simulink model "Fly_By_Wire_Component_Architecture"  (R2025a)
settings: Solver=VariableStepAuto  StartTime=0.0  StopTime=10.0  RelTol=1e-3
settings Model: Creator=kmara  LastModifiedBy=annic

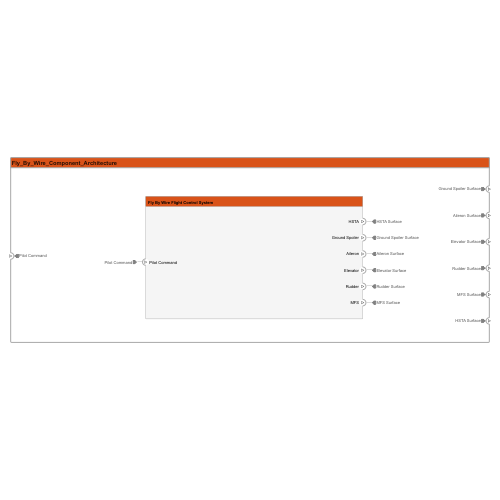
[thumbnail: Simulink's stored preview of the top-level diagram]
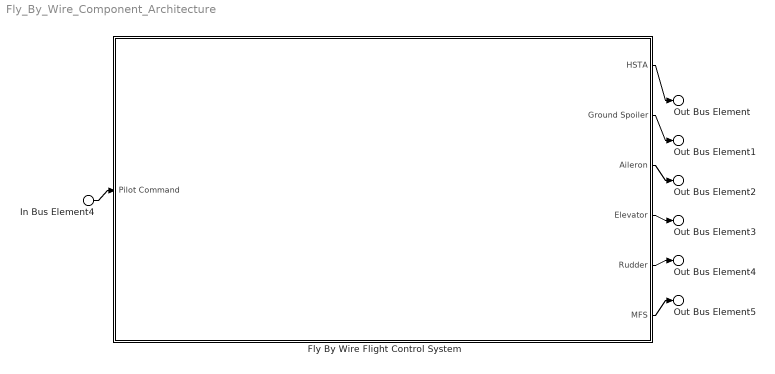
== system Fly_By_Wire_Component_Architecture ==
  In Bus Element4 : Inport  PortName=Pilot Command
  Fly By Wire Flight Control System : Subsystem
      settings: PortSchema="{\"entries\":[{\"content\":{\"headerSize\":26,\"margin\":15,\"minimumSpacing\":25,\"sides\":[{\"content\":{\"connectorIds\":[\"In1\"]},\"type\":\"ConnectorPlacement.EquallySpacedRectSide\",\"uuid\":\"7c02a101-dcdb-4ce7-aa42-618b1352dc14\"},{\"content\":{\"connectorIds\":[\"Out1\",\"Out2\",\"Out3\",\"Out4\",\"Out5\",\"Out6\"],\"side\":\"RIGHT\"},\"type\":\"ConnectorPlacement.EquallySpacedRectSide\",\"uuid\":\"7a5c8ca0-4377-40e0-b018-2d4752105c97\"},{\"content\":{\"side\":\"TOP\"},\"type\":\"ConnectorPlacement.EquallySpacedRectSide\",\"uuid\":\"1a585cfa-94cd-4fa4-8da7-05bff58353c8\"}]},\"type\":\"ConnectorPlacement.EquallySpacedConnector\",\"uuid\":\"b5a72803-1929-44a1-ac0b-19b19b30c1d3\"}],\"packageUris\":[\"http://schema.mathworks.com/mf0/Connector/R2020b\"],\"version\":\"1.0\"}"
  Out Bus Element1 : Outport  PortName=Ground Spoiler Surface
  Out Bus Element2 : Outport  Port=2  PortName=Aileron Surface
  Out Bus Element3 : Outport  Port=3  PortName=Elevator Surface
  Out Bus Element4 : Outport  Port=4  PortName=Rudder Surface
  Out Bus Element5 : Outport  Port=5  PortName=MFS Surface
  Out Bus Element : Outport  Port=6  PortName=HSTA Surface
  wires:
  Fly By Wire Flight Control System/1(HSTA) -> Out Bus Element/1
  Fly By Wire Flight Control System/2(Ground Spoiler) -> Out Bus Element1/1
  Fly By Wire Flight Control System/3(Aileron) -> Out Bus Element2/1
  Fly By Wire Flight Control System/4(Elevator) -> Out Bus Element3/1
  Fly By Wire Flight Control System/5(Rudder) -> Out Bus Element4/1
  Fly By Wire Flight Control System/6(MFS) -> Out Bus Element5/1
  In Bus Element4/1 -> Fly By Wire Flight Control System/1(Pilot Command)

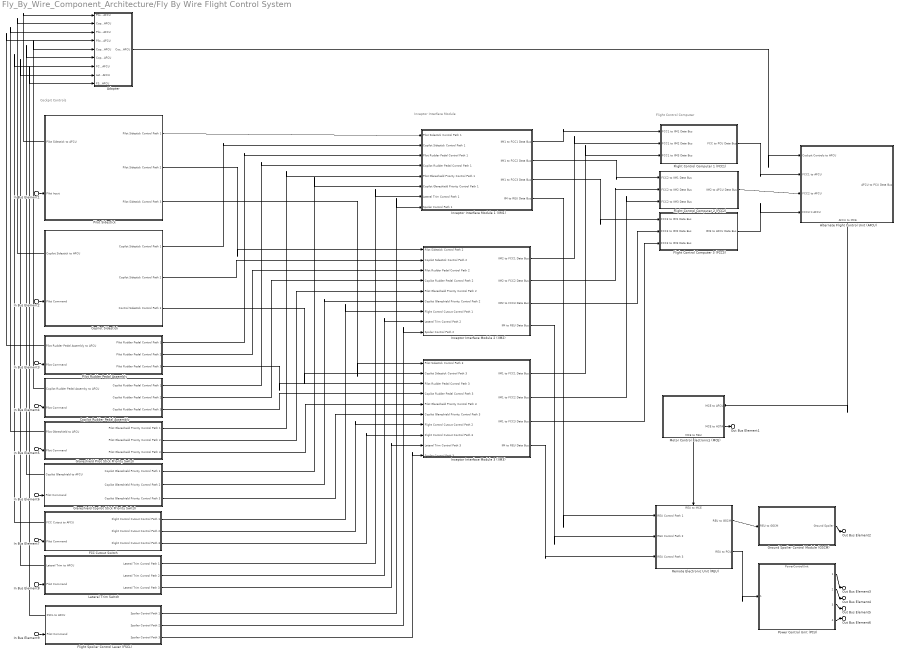
== system Fly_By_Wire_Component_Architecture/Fly By Wire Flight Control System ==
  note: Inceptor Interface Module
  note: Flight Control Computer
  note: Cockpit Controls
  In Bus Element{1..9} (9 alike) : Inport  PortName=Pilot Command
  Adapter : Subsystem
      settings: PortSchema="{\"entries\":[{\"content\":{\"margin\":10,\"minimumSpacing\":15,\"sides\":[{\"content\":{\"connectorIds\":[\"In9\",\"In2\",\"In1\",\"In3\",\"In4\",\"In5\",\"In6\",\"In7\",\"In8\"]},\"type\":\"ConnectorPlacement.EquallySpacedRectSide\",\"uuid\":\"7c02a101-dcdb-4ce7-aa42-618b1352dc14\"},{\"content\":{\"connectorIds\":[\"Out1\"],\"side\":\"RIGHT\"},\"type\":\"ConnectorPlacement.EquallySpacedRectSide\",\"uuid\":\"7a5c8ca0-4377-40e0-b018-2d4752105c97\"},{\"content\":{\"side\":\"TOP\"},\"type\":\"ConnectorPlacement.EquallySpacedRectSide\",\"uuid\":\"1a585cfa-94cd-4fa4-8da7-05bff58353c8\"},{\"content\":{\"side\":\"BOTTOM\"},\"type\":\"ConnectorPlacement.EquallySpacedRectSide\",\"uuid\":\"bc495dab-060b-4ff9-9574-e388694fe188\"}]},\"type\":\"ConnectorPlacement.EquallySpacedConnector\",\"uuid\":\"b5a72803-1929-44a1-ac0b-19b19b30c1d3\"}],\"packageUris\":[\"http://schema.mathworks.com/mf0/Connector/R2020b\"],\"version\":\"1.0\"}"
  Alternate Flight Control Unit (AFCU) : Subsystem
      settings: PortSchema="{\"entries\":[{\"content\":{\"headerSize\":26,\"margin\":15,\"minimumSpacing\":25,\"sides\":[{\"content\":{\"connectorIds\":[\"In1\",\"In2\",\"In3\",\"In4\"]},\"type\":\"ConnectorPlacement.EquallySpacedRectSide\",\"uuid\":\"76a6f17d-cf4a-44f4-8892-601f52e19bd9\"},{\"content\":{\"connectorIds\":[\"Out2\"],\"side\":\"RIGHT\"},\"type\":\"ConnectorPlacement.EquallySpacedRectSide\",\"uuid\":\"5dcbb71c-e863-4861-a43d-ad9fb4188728\"},{\"content\":{\"side\":\"TOP\"},\"type\":\"ConnectorPlacement.EquallySpacedRectSide\",\"uuid\":\"68738236-1483-402e-9d85-5d65cc06fd90\"},{\"content\":{\"connectorIds\":[\"Out1\"],\"side\":\"BOTTOM\"},\"type\":\"ConnectorPlacement.EquallySpacedRectSide\",\"uuid\":\"9a083ef4-6723-4d8e-ad60-e307f1dd41e6\"}]},\"type\":\"ConnectorPlacement.EquallySpacedConnector\",\"uuid\":\"56deb81c-b974-4059-9f73-f14d44365067\"}],\"packageUris\":[\"http://schema.mathworks.com/mf0/Connector/R2020b\"],\"version\":\"1.0\"}"
  Copilot Rudder Pedal Assembly : Subsystem
      settings: PortSchema="{\"entries\":[{\"content\":{\"headerSize\":26,\"margin\":15,\"minimumSpacing\":25,\"sides\":[{\"content\":{\"connectorIds\":[\"Out1\",\"In1\"]},\"type\":\"ConnectorPlacement.EquallySpacedRectSide\",\"uuid\":\"76a6f17d-cf4a-44f4-8892-601f52e19bd9\"},{\"content\":{\"connectorIds\":[\"Out2\",\"Out3\",\"Out4\"],\"side\":\"RIGHT\"},\"type\":\"ConnectorPlacement.EquallySpacedRectSide\",\"uuid\":\"5dcbb71c-e863-4861-a43d-ad9fb4188728\"},{\"content\":{\"side\":\"TOP\"},\"type\":\"ConnectorPlacement.EquallySpacedRectSide\",\"uuid\":\"68738236-1483-402e-9d85-5d65cc06fd90\"}]},\"type\":\"ConnectorPlacement.EquallySpacedConnector\",\"uuid\":\"56deb81c-b974-4059-9f73-f14d44365067\"}],\"packageUris\":[\"http://schema.mathworks.com/mf0/Connector/R2020b\"],\"version\":\"1.0\"}"
  Copilot Sidestick : Subsystem
      settings: PortSchema="{\"entries\":[{\"content\":{\"headerSize\":26,\"margin\":15,\"minimumSpacing\":25,\"sides\":[{\"content\":{\"connectorIds\":[\"Out1\",\"In1\"]},\"type\":\"ConnectorPlacement.EquallySpacedRectSide\",\"uuid\":\"76a6f17d-cf4a-44f4-8892-601f52e19bd9\"},{\"content\":{\"connectorIds\":[\"Out2\",\"Out3\",\"Out4\"],\"side\":\"RIGHT\"},\"type\":\"ConnectorPlacement.EquallySpacedRectSide\",\"uuid\":\"5dcbb71c-e863-4861-a43d-ad9fb4188728\"},{\"content\":{\"side\":\"TOP\"},\"type\":\"ConnectorPlacement.EquallySpacedRectSide\",\"uuid\":\"68738236-1483-402e-9d85-5d65cc06fd90\"}]},\"type\":\"ConnectorPlacement.EquallySpacedConnector\",\"uuid\":\"56deb81c-b974-4059-9f73-f14d44365067\"}],\"packageUris\":[\"http://schema.mathworks.com/mf0/Connector/R2020b\"],\"version\":\"1.0\"}"
  FCC Cutout Switch : Subsystem
      settings: PortSchema="{\"entries\":[{\"content\":{\"headerSize\":26,\"margin\":15,\"minimumSpacing\":25,\"sides\":[{\"content\":{\"connectorIds\":[\"Out1\",\"In1\"]},\"type\":\"ConnectorPlacement.EquallySpacedRectSide\",\"uuid\":\"76a6f17d-cf4a-44f4-8892-601f52e19bd9\"},{\"content\":{\"connectorIds\":[\"Out2\",\"Out3\",\"Out4\"],\"side\":\"RIGHT\"},\"type\":\"ConnectorPlacement.EquallySpacedRectSide\",\"uuid\":\"5dcbb71c-e863-4861-a43d-ad9fb4188728\"},{\"content\":{\"side\":\"TOP\"},\"type\":\"ConnectorPlacement.EquallySpacedRectSide\",\"uuid\":\"68738236-1483-402e-9d85-5d65cc06fd90\"}]},\"type\":\"ConnectorPlacement.EquallySpacedConnector\",\"uuid\":\"56deb81c-b974-4059-9f73-f14d44365067\"}],\"packageUris\":[\"http://schema.mathworks.com/mf0/Connector/R2020b\"],\"version\":\"1.0\"}"
  Flight Control Computer 1 (FCC1) : Subsystem
      settings: PortSchema="{\"entries\":[{\"content\":{\"headerSize\":26,\"margin\":15,\"minimumSpacing\":25,\"sides\":[{\"content\":{\"connectorIds\":[\"In1\",\"In2\",\"In3\"]},\"type\":\"ConnectorPlacement.EquallySpacedRectSide\",\"uuid\":\"76a6f17d-cf4a-44f4-8892-601f52e19bd9\"},{\"content\":{\"connectorIds\":[\"Out1\"],\"side\":\"RIGHT\"},\"type\":\"ConnectorPlacement.EquallySpacedRectSide\",\"uuid\":\"5dcbb71c-e863-4861-a43d-ad9fb4188728\"},{\"content\":{\"side\":\"TOP\"},\"type\":\"ConnectorPlacement.EquallySpacedRectSide\",\"uuid\":\"68738236-1483-402e-9d85-5d65cc06fd90\"}]},\"type\":\"ConnectorPlacement.EquallySpacedConnector\",\"uuid\":\"56deb81c-b974-4059-9f73-f14d44365067\"}],\"packageUris\":[\"http://schema.mathworks.com/mf0/Connector/R2020b\"],\"version\":\"1.0\"}"
  Flight Control Computer 2 (FCC2) : Subsystem
      settings: PortSchema="{\"entries\":[{\"content\":{\"headerSize\":26,\"margin\":15,\"minimumSpacing\":25,\"sides\":[{\"content\":{\"connectorIds\":[\"In1\",\"In2\",\"In3\"]},\"type\":\"ConnectorPlacement.EquallySpacedRectSide\",\"uuid\":\"3265125f-5582-4687-bb7d-dadd2bb28ee5\"},{\"content\":{\"connectorIds\":[\"Out1\"],\"side\":\"RIGHT\"},\"type\":\"ConnectorPlacement.EquallySpacedRectSide\",\"uuid\":\"e765b43a-7d93-4967-9a71-e180bcccebcf\"},{\"content\":{\"side\":\"TOP\"},\"type\":\"ConnectorPlacement.EquallySpacedRectSide\",\"uuid\":\"6eb4b4e6-82d4-477f-9521-c512acf3f79c\"}]},\"type\":\"ConnectorPlacement.EquallySpacedConnector\",\"uuid\":\"cacda304-df90-44d5-b969-56e5837c68bb\"}],\"packageUris\":[\"http://schema.mathworks.com/mf0/Connector/R2020b\"],\"version\":\"1.0\"}"
  Flight Control Computer 3 (FCC3) : Subsystem
      settings: PortSchema="{\"entries\":[{\"content\":{\"headerSize\":26,\"margin\":15,\"minimumSpacing\":25,\"sides\":[{\"content\":{\"connectorIds\":[\"In1\",\"In2\",\"In3\"]},\"type\":\"ConnectorPlacement.EquallySpacedRectSide\",\"uuid\":\"3265125f-5582-4687-bb7d-dadd2bb28ee5\"},{\"content\":{\"connectorIds\":[\"Out1\"],\"side\":\"RIGHT\"},\"type\":\"ConnectorPlacement.EquallySpacedRectSide\",\"uuid\":\"e765b43a-7d93-4967-9a71-e180bcccebcf\"},{\"content\":{\"side\":\"TOP\"},\"type\":\"ConnectorPlacement.EquallySpacedRectSide\",\"uuid\":\"6eb4b4e6-82d4-477f-9521-c512acf3f79c\"}]},\"type\":\"ConnectorPlacement.EquallySpacedConnector\",\"uuid\":\"cacda304-df90-44d5-b969-56e5837c68bb\"}],\"packageUris\":[\"http://schema.mathworks.com/mf0/Connector/R2020b\"],\"version\":\"1.0\"}"
  Flight Spoiler Control Lever (FSCL) : Subsystem
      settings: PortSchema="{\"entries\":[{\"content\":{\"headerSize\":26,\"margin\":15,\"minimumSpacing\":25,\"sides\":[{\"content\":{\"connectorIds\":[\"Out1\",\"In1\"]},\"type\":\"ConnectorPlacement.EquallySpacedRectSide\",\"uuid\":\"76a6f17d-cf4a-44f4-8892-601f52e19bd9\"},{\"content\":{\"connectorIds\":[\"Out2\",\"Out3\",\"Out4\"],\"side\":\"RIGHT\"},\"type\":\"ConnectorPlacement.EquallySpacedRectSide\",\"uuid\":\"5dcbb71c-e863-4861-a43d-ad9fb4188728\"},{\"content\":{\"side\":\"TOP\"},\"type\":\"ConnectorPlacement.EquallySpacedRectSide\",\"uuid\":\"68738236-1483-402e-9d85-5d65cc06fd90\"}]},\"type\":\"ConnectorPlacement.EquallySpacedConnector\",\"uuid\":\"56deb81c-b974-4059-9f73-f14d44365067\"}],\"packageUris\":[\"http://schema.mathworks.com/mf0/Connector/R2020b\"],\"version\":\"1.0\"}"
  Glareshield Copilot Stick Priority Switch : Subsystem
      settings: PortSchema="{\"entries\":[{\"content\":{\"headerSize\":26,\"margin\":15,\"minimumSpacing\":25,\"sides\":[{\"content\":{\"connectorIds\":[\"Out1\",\"In1\"]},\"type\":\"ConnectorPlacement.EquallySpacedRectSide\",\"uuid\":\"76a6f17d-cf4a-44f4-8892-601f52e19bd9\"},{\"content\":{\"connectorIds\":[\"Out2\",\"Out3\",\"Out4\"],\"side\":\"RIGHT\"},\"type\":\"ConnectorPlacement.EquallySpacedRectSide\",\"uuid\":\"5dcbb71c-e863-4861-a43d-ad9fb4188728\"},{\"content\":{\"side\":\"TOP\"},\"type\":\"ConnectorPlacement.EquallySpacedRectSide\",\"uuid\":\"68738236-1483-402e-9d85-5d65cc06fd90\"}]},\"type\":\"ConnectorPlacement.EquallySpacedConnector\",\"uuid\":\"56deb81c-b974-4059-9f73-f14d44365067\"}],\"packageUris\":[\"http://schema.mathworks.com/mf0/Connector/R2020b\"],\"version\":\"1.0\"}"
  Glareshield Pilot Stick Priority Switch : Subsystem
      settings: PortSchema="{\"entries\":[{\"content\":{\"headerSize\":26,\"margin\":15,\"minimumSpacing\":25,\"sides\":[{\"content\":{\"connectorIds\":[\"Out1\",\"In1\"]},\"type\":\"ConnectorPlacement.EquallySpacedRectSide\",\"uuid\":\"76a6f17d-cf4a-44f4-8892-601f52e19bd9\"},{\"content\":{\"connectorIds\":[\"Out2\",\"Out3\",\"Out4\"],\"side\":\"RIGHT\"},\"type\":\"ConnectorPlacement.EquallySpacedRectSide\",\"uuid\":\"5dcbb71c-e863-4861-a43d-ad9fb4188728\"},{\"content\":{\"side\":\"TOP\"},\"type\":\"ConnectorPlacement.EquallySpacedRectSide\",\"uuid\":\"68738236-1483-402e-9d85-5d65cc06fd90\"}]},\"type\":\"ConnectorPlacement.EquallySpacedConnector\",\"uuid\":\"56deb81c-b974-4059-9f73-f14d44365067\"}],\"packageUris\":[\"http://schema.mathworks.com/mf0/Connector/R2020b\"],\"version\":\"1.0\"}"
  Ground Spoiler Control Module (GSCM) : Subsystem
      settings: PortSchema="{\"entries\":[{\"content\":{\"headerSize\":26,\"margin\":15,\"minimumSpacing\":25,\"sides\":[{\"content\":{\"connectorIds\":[\"In1\"]},\"type\":\"ConnectorPlacement.EquallySpacedRectSide\",\"uuid\":\"76a6f17d-cf4a-44f4-8892-601f52e19bd9\"},{\"content\":{\"connectorIds\":[\"Out1\"],\"side\":\"RIGHT\"},\"type\":\"ConnectorPlacement.EquallySpacedRectSide\",\"uuid\":\"5dcbb71c-e863-4861-a43d-ad9fb4188728\"},{\"content\":{\"side\":\"TOP\"},\"type\":\"ConnectorPlacement.EquallySpacedRectSide\",\"uuid\":\"68738236-1483-402e-9d85-5d65cc06fd90\"}]},\"type\":\"ConnectorPlacement.EquallySpacedConnector\",\"uuid\":\"56deb81c-b974-4059-9f73-f14d44365067\"}],\"packageUris\":[\"http://schema.mathworks.com/mf0/Connector/R2020b\"],\"version\":\"1.0\"}"
  Inceptor Interface Module 1 (IIM1) : Subsystem
      settings: PortSchema="{\"entries\":[{\"content\":{\"headerSize\":26,\"margin\":15,\"minimumSpacing\":25,\"sides\":[{\"content\":{\"connectorIds\":[\"In1\",\"In2\",\"In3\",\"In4\",\"In5\",\"In6\",\"In7\",\"In8\"]},\"type\":\"ConnectorPlacement.EquallySpacedRectSide\",\"uuid\":\"76a6f17d-cf4a-44f4-8892-601f52e19bd9\"},{\"content\":{\"connectorIds\":[\"Out1\",\"Out2\",\"Out3\",\"Out4\"],\"side\":\"RIGHT\"},\"type\":\"ConnectorPlacement.EquallySpacedRectSide\",\"uuid\":\"5dcbb71c-e863-4861-a43d-ad9fb4188728\"},{\"content\":{\"side\":\"TOP\"},\"type\":\"ConnectorPlacement.EquallySpacedRectSide\",\"uuid\":\"68738236-1483-402e-9d85-5d65cc06fd90\"},{\"content\":{\"side\":\"BOTTOM\"},\"type\":\"ConnectorPlacement.EquallySpacedRectSide\",\"uuid\":\"f9a83800-3852-40cb-9c1f-6e0812a46961\"}]},\"type\":\"ConnectorPlacement.EquallySpacedConnector\",\"uuid\":\"56deb81c-b974-4059-9f73-f14d44365067\"}],\"packageUris\":[\"http://schema.mathworks.com/mf0/Connector/R2020b\"],\"version\":\"1.0\"}"
  Inceptor Interface Module 2 (IIM2) : Subsystem
      settings: PortSchema="{\"entries\":[{\"content\":{\"headerSize\":26,\"margin\":15,\"minimumSpacing\":25,\"sides\":[{\"content\":{\"connectorIds\":[\"In1\",\"In3\",\"In2\",\"In4\",\"In5\",\"In6\",\"In7\",\"In8\",\"In9\"]},\"type\":\"ConnectorPlacement.EquallySpacedRectSide\",\"uuid\":\"76a6f17d-cf4a-44f4-8892-601f52e19bd9\"},{\"content\":{\"connectorIds\":[\"Out1\",\"Out2\",\"Out3\",\"Out4\"],\"side\":\"RIGHT\"},\"type\":\"ConnectorPlacement.EquallySpacedRectSide\",\"uuid\":\"5dcbb71c-e863-4861-a43d-ad9fb4188728\"},{\"content\":{\"side\":\"TOP\"},\"type\":\"ConnectorPlacement.EquallySpacedRectSide\",\"uuid\":\"68738236-1483-402e-9d85-5d65cc06fd90\"},{\"content\":{\"side\":\"BOTTOM\"},\"type\":\"ConnectorPlacement.EquallySpacedRectSide\",\"uuid\":\"f9a83800-3852-40cb-9c1f-6e0812a46961\"}]},\"type\":\"ConnectorPlacement.EquallySpacedConnector\",\"uuid\":\"56deb81c-b974-4059-9f73-f14d44365067\"}],\"packageUris\":[\"http://schema.mathworks.com/mf0/Connector/R2020b\"],\"version\":\"1.0\"}"
  Inceptor Interface Module 3 (IIM3) : Subsystem
      settings: PortSchema="{\"entries\":[{\"content\":{\"headerSize\":26,\"margin\":15,\"minimumSpacing\":25,\"sides\":[{\"content\":{\"connectorIds\":[\"In1\",\"In2\",\"In3\",\"In4\",\"In5\",\"In6\",\"In7\",\"In8\",\"In9\",\"In10\"]},\"type\":\"ConnectorPlacement.EquallySpacedRectSide\",\"uuid\":\"76a6f17d-cf4a-44f4-8892-601f52e19bd9\"},{\"content\":{\"connectorIds\":[\"Out1\",\"Out2\",\"Out3\",\"Out4\"],\"side\":\"RIGHT\"},\"type\":\"ConnectorPlacement.EquallySpacedRectSide\",\"uuid\":\"5dcbb71c-e863-4861-a43d-ad9fb4188728\"},{\"content\":{\"side\":\"TOP\"},\"type\":\"ConnectorPlacement.EquallySpacedRectSide\",\"uuid\":\"68738236-1483-402e-9d85-5d65cc06fd90\"},{\"content\":{\"side\":\"BOTTOM\"},\"type\":\"ConnectorPlacement.EquallySpacedRectSide\",\"uuid\":\"f9a83800-3852-40cb-9c1f-6e0812a46961\"}]},\"type\":\"ConnectorPlacement.EquallySpacedConnector\",\"uuid\":\"56deb81c-b974-4059-9f73-f14d44365067\"}],\"packageUris\":[\"http://schema.mathworks.com/mf0/Connector/R2020b\"],\"version\":\"1.0\"}"
  Lateral Trim Switch : Subsystem
      settings: PortSchema="{\"entries\":[{\"content\":{\"headerSize\":26,\"margin\":15,\"minimumSpacing\":25,\"sides\":[{\"content\":{\"connectorIds\":[\"Out1\",\"In1\"]},\"type\":\"ConnectorPlacement.EquallySpacedRectSide\",\"uuid\":\"76a6f17d-cf4a-44f4-8892-601f52e19bd9\"},{\"content\":{\"connectorIds\":[\"Out2\",\"Out3\",\"Out4\"],\"side\":\"RIGHT\"},\"type\":\"ConnectorPlacement.EquallySpacedRectSide\",\"uuid\":\"5dcbb71c-e863-4861-a43d-ad9fb4188728\"},{\"content\":{\"side\":\"TOP\"},\"type\":\"ConnectorPlacement.EquallySpacedRectSide\",\"uuid\":\"68738236-1483-402e-9d85-5d65cc06fd90\"}]},\"type\":\"ConnectorPlacement.EquallySpacedConnector\",\"uuid\":\"56deb81c-b974-4059-9f73-f14d44365067\"}],\"packageUris\":[\"http://schema.mathworks.com/mf0/Connector/R2020b\"],\"version\":\"1.0\"}"
  Motor Control Electronics (MCE) : Subsystem
      settings: PortSchema="{\"entries\":[{\"content\":{\"headerSize\":26,\"margin\":15,\"minimumSpacing\":25,\"sides\":[{\"content\":{},\"type\":\"ConnectorPlacement.EquallySpacedRectSide\",\"uuid\":\"7c02a101-dcdb-4ce7-aa42-618b1352dc14\"},{\"content\":{\"connectorIds\":[\"In1\",\"Out1\"],\"side\":\"RIGHT\"},\"type\":\"ConnectorPlacement.EquallySpacedRectSide\",\"uuid\":\"7a5c8ca0-4377-40e0-b018-2d4752105c97\"},{\"content\":{\"side\":\"TOP\"},\"type\":\"ConnectorPlacement.EquallySpacedRectSide\",\"uuid\":\"1a585cfa-94cd-4fa4-8da7-05bff58353c8\"},{\"content\":{\"connectorIds\":[\"Out2\"],\"side\":\"BOTTOM\"},\"type\":\"ConnectorPlacement.EquallySpacedRectSide\",\"uuid\":\"a4e30391-3178-49c1-81f8-9566370a7e69\"}]},\"type\":\"ConnectorPlacement.EquallySpacedConnector\",\"uuid\":\"b5a72803-1929-44a1-ac0b-19b19b30c1d3\"}],\"packageUris\":[\"http://schema.mathworks.com/mf0/Connector/R2020b\"],\"version\":\"1.0\"}"
  Pilot Rudder Pedal Assembly : Subsystem
      settings: PortSchema="{\"entries\":[{\"content\":{\"headerSize\":26,\"margin\":15,\"minimumSpacing\":25,\"sides\":[{\"content\":{\"connectorIds\":[\"Out1\",\"In1\"]},\"type\":\"ConnectorPlacement.EquallySpacedRectSide\",\"uuid\":\"76a6f17d-cf4a-44f4-8892-601f52e19bd9\"},{\"content\":{\"connectorIds\":[\"Out2\",\"Out4\",\"Out3\"],\"side\":\"RIGHT\"},\"type\":\"ConnectorPlacement.EquallySpacedRectSide\",\"uuid\":\"5dcbb71c-e863-4861-a43d-ad9fb4188728\"},{\"content\":{\"side\":\"TOP\"},\"type\":\"ConnectorPlacement.EquallySpacedRectSide\",\"uuid\":\"68738236-1483-402e-9d85-5d65cc06fd90\"}]},\"type\":\"ConnectorPlacement.EquallySpacedConnector\",\"uuid\":\"56deb81c-b974-4059-9f73-f14d44365067\"}],\"packageUris\":[\"http://schema.mathworks.com/mf0/Connector/R2020b\"],\"version\":\"1.0\"}"
  Pilot Sidestick : Subsystem
      settings: PortSchema="{\"entries\":[{\"content\":{\"headerSize\":26,\"margin\":15,\"minimumSpacing\":25,\"sides\":[{\"content\":{\"connectorIds\":[\"Out4\",\"In1\"]},\"type\":\"ConnectorPlacement.EquallySpacedRectSide\",\"uuid\":\"76a6f17d-cf4a-44f4-8892-601f52e19bd9\"},{\"content\":{\"connectorIds\":[\"Out1\",\"Out2\",\"Out3\"],\"side\":\"RIGHT\"},\"type\":\"ConnectorPlacement.EquallySpacedRectSide\",\"uuid\":\"5dcbb71c-e863-4861-a43d-ad9fb4188728\"},{\"content\":{\"side\":\"TOP\"},\"type\":\"ConnectorPlacement.EquallySpacedRectSide\",\"uuid\":\"68738236-1483-402e-9d85-5d65cc06fd90\"}]},\"type\":\"ConnectorPlacement.EquallySpacedConnector\",\"uuid\":\"56deb81c-b974-4059-9f73-f14d44365067\"}],\"packageUris\":[\"http://schema.mathworks.com/mf0/Connector/R2020b\"],\"version\":\"1.0\"}"
  Power Control Unit (PCU) : ModelReference  ModelNameDialog=PowerControlUnit  SimulationMode=Normal  ModelReferenceVersion=3.0
      settings: PortSchema="{\"entries\":[{\"content\":{\"headerSize\":38,\"margin\":15,\"minimumSpacing\":25,\"sides\":[{\"content\":{\"connectorIds\":[\"In1\"]},\"type\":\"ConnectorPlacement.EquallySpacedRectSide\",\"uuid\":\"b5cc4046-2a7b-4e82-a24e-8f0b5fbe8f3b\"},{\"content\":{\"connectorIds\":[\"Out1\",\"Out2\",\"Out3\",\"Out4\"],\"side\":\"RIGHT\"},\"type\":\"ConnectorPlacement.EquallySpacedRectSide\",\"uuid\":\"a37fb25c-992f-4dee-9f4d-cb05ec6d06aa\"},{\"content\":{\"side\":\"TOP\"},\"type\":\"ConnectorPlacement.EquallySpacedRectSide\",\"uuid\":\"6865807b-cb28-45bc-8645-e4c4882f3eb7\"}]},\"type\":\"ConnectorPlacement.EquallySpacedConnector\",\"uuid\":\"a108b503-ea1d-46cf-b1fa-be423a2d8416\"}],\"packageUris\":[\"http://schema.mathworks.com/mf0/Connector/R2020b\"],\"version\":\"1.0\"}"
  Remote Electronic Unit (REU) : Subsystem
      settings: PortSchema="{\"entries\":[{\"content\":{\"headerSize\":26,\"margin\":15,\"minimumSpacing\":25,\"sides\":[{\"content\":{\"connectorIds\":[\"In2\",\"In3\",\"In4\"]},\"type\":\"ConnectorPlacement.EquallySpacedRectSide\",\"uuid\":\"76a6f17d-cf4a-44f4-8892-601f52e19bd9\"},{\"content\":{\"connectorIds\":[\"Out1\",\"Out2\"],\"side\":\"RIGHT\"},\"type\":\"ConnectorPlacement.EquallySpacedRectSide\",\"uuid\":\"5dcbb71c-e863-4861-a43d-ad9fb4188728\"},{\"content\":{\"connectorIds\":[\"In1\"],\"side\":\"TOP\"},\"type\":\"ConnectorPlacement.EquallySpacedRectSide\",\"uuid\":\"68738236-1483-402e-9d85-5d65cc06fd90\"},{\"content\":{\"side\":\"BOTTOM\"},\"type\":\"ConnectorPlacement.EquallySpacedRectSide\",\"uuid\":\"ca264cd1-95f3-4bee-bece-6d79b6f7bd38\"}]},\"type\":\"ConnectorPlacement.EquallySpacedConnector\",\"uuid\":\"56deb81c-b974-4059-9f73-f14d44365067\"}],\"packageUris\":[\"http://schema.mathworks.com/mf0/Connector/R2020b\"],\"version\":\"1.0\"}"
  Out Bus Element1 : Outport  PortName=HSTA
  Out Bus Element2 : Outport  Port=2  PortName=Ground Spoiler
  Out Bus Element3 : Outport  Port=3  PortName=Aileron
  Out Bus Element4 : Outport  Port=4  PortName=Elevator
  Out Bus Element5 : Outport  Port=5  PortName=Rudder
  Out Bus Element6 : Outport  Port=6  PortName=MFS
  wires:
  In Bus Element7/1 -> FCC Cutout Switch/1(Pilot Command)
  In Bus Element2/1 -> Copilot Sidestick/1(Pilot Command)
  Motor Control Electronics (MCE)/1(MCE to HSTA) -> Out Bus Element1/1
  Alternate Flight Control Unit (AFCU)/1(AFCU to MCE) -> Motor Control Electronics (MCE)/1(MCE to AFCU)
  Motor Control Electronics (MCE)/2(MCE to REU) -> Remote Electronic Unit (REU)/1(REU to MCE)
  FCC Cutout Switch/1(FCC Cutout to AFCU) -> Adapter/6(FCC Cutout to AFCU)
  Flight Spoiler Control Lever (FSCL)/1(FSCL to AFCU) -> Adapter/8(FSCL to AFCU)
  Remote Electronic Unit (REU)/1(REU to GSCM) -> Ground Spoiler Control Module (GSCM)/1(REU to GSCM)
  Pilot Sidestick/1(Pilot Sidestick Control Path 1) -> Inceptor Interface Module 1 (IIM1)/1(Pilot Sidestick Control Path 1)
  Ground Spoiler Control Module (GSCM)/1(Ground Spoiler) -> Out Bus Element2/1
  Copilot Rudder Pedal Assembly/3(Copilot Rudder Pedal Control Path 2) -> Inceptor Interface Module 2 (IIM2)/4(Copilot Rudder Pedal Control Path 2)
  Lateral Trim Switch/1(Lateral Trim to AFCU) -> Adapter/7(Lateral Trim to AFCU)
  Flight Control Computer 1 (FCC1)/1(FCC to PCU Data Bus) -> Alternate Flight Control Unit (AFCU)/2(FCC1 to AFCU)
  In Bus Element9/1 -> Flight Spoiler Control Lever (FSCL)/1(Pilot Command)
  FCC Cutout Switch/2(Flight Control Cutout Control Path 1) -> Inceptor Interface Module 2 (IIM2)/7(Flight Control Cutout Control Path 1)
  Lateral Trim Switch/3(Lateral Trim Control Path 2) -> Inceptor Interface Module 2 (IIM2)/8(Lateral Trim Control Path 2)
  Inceptor Interface Module 3 (IIM3)/2(IIM1 to FCC2 Data Bus) -> Flight Control Computer 2 (FCC2)/3(FCC2 to IIM3 Data Bus)
  Pilot Sidestick/2("Pilot Sidestick Control Path 2 ") -> Inceptor Interface Module 2 (IIM2)/1("Pilot Sidestick Control Path 2 ")
  Glareshield Copilot Stick Priority Switch/2(Copilot Glareshield Priority Control Path 1) -> Inceptor Interface Module 1 (IIM1)/6(Copilot Glareshield Priority Control Path 1)
  Flight Spoiler Control Lever (FSCL)/2(Spoiler Control Path 1) -> Inceptor Interface Module 1 (IIM1)/8(Spoiler Control Path 1)
  Pilot Sidestick/3(Pilot Sidestick Control Path 3) -> Inceptor Interface Module 3 (IIM3)/1("Pilot Sidestick Control Path 3 ")
  Flight Control Computer 2 (FCC2)/1(IIM2 to AFCU Data Bus) -> Alternate Flight Control Unit (AFCU)/3(FCC2 to AFCU)
  Lateral Trim Switch/4(Lateral Trim Control Path 3) -> Inceptor Interface Module 3 (IIM3)/9(Lateral Trim Control Path 3)
  Pilot Rudder Pedal Assembly/4(Pilot Rudder Pedal Control Path 2) -> Inceptor Interface Module 2 (IIM2)/2(Pilot Rudder Pedal Control Path 2)
  Copilot Sidestick/2(Copilot Sidestick Control Path 1) -> Inceptor Interface Module 1 (IIM1)/2(Copilot Sidestick Control Path 1)
  Glareshield Copilot Stick Priority Switch/4(Copilot Glareshield Priority Control Path 3) -> Inceptor Interface Module 3 (IIM3)/6(Copilot Glareshield Priority Control Path 3)
  Glareshield Copilot Stick Priority Switch/3(Copilot Glareshield Priority Control Path 2) -> Inceptor Interface Module 2 (IIM2)/6(Copilot Glareshield Priority Control Path 2)
  Glareshield Pilot Stick Priority Switch/3(Pilot Glareshield Priority Control Path 2) -> Inceptor Interface Module 2 (IIM2)/5(Pilot Glareshield Priority Control Path 2)
  Flight Spoiler Control Lever (FSCL)/4(Spoiler Control Path 3) -> Inceptor Interface Module 3 (IIM3)/10(Spoiler Control Path 3)
  Inceptor Interface Module 1 (IIM1)/2(IIM1 to FCC2 Data Bus) -> Flight Control Computer 2 (FCC2)/1(FCC2 to IIM1 Data Bus)
  Inceptor Interface Module 2 (IIM2)/1(IIM2 to FCC1 Data Bus) -> Flight Control Computer 1 (FCC1)/2(FCC1 to IIM2 Data Bus)
  Inceptor Interface Module 1 (IIM1)/3(IIM1 to FCC3 Data Bus) -> Flight Control Computer 3 (FCC3)/1(FCC3 to IIM1 Data Bus)
  Pilot Rudder Pedal Assembly/2(Pilot Rudder Pedal Control Path 1) -> Inceptor Interface Module 1 (IIM1)/3(Pilot Rudder Pedal Control Path 1)
  Copilot Sidestick/4(Control Sidestick Control Path 3) -> Inceptor Interface Module 3 (IIM3)/2(Copilot Sidestick Control Path 3)
  Inceptor Interface Module 1 (IIM1)/1(IIM1 to FCC1 Data Bus) -> Flight Control Computer 1 (FCC1)/1(FCC1 to IIM1 Data Bus)
  Copilot Sidestick/1(Copilot Sidestick to AFCU) -> Adapter/2(Copilot Sidestick to AFCU)
  FCC Cutout Switch/3(Flight Control Cutout Control Path 2) -> Inceptor Interface Module 3 (IIM3)/7(Flight Control Cutout Control Path 2)
  Inceptor Interface Module 2 (IIM2)/4(IIM to REU Data Bus) -> Remote Electronic Unit (REU)/3(REU Control Path 2)
  Flight Spoiler Control Lever (FSCL)/3(Spoiler Control Path 2) -> Inceptor Interface Module 2 (IIM2)/9(Spoiler Control Path 2)
  Glareshield Copilot Stick Priority Switch/1(Copilot Glareshield to AFCU) -> Adapter/5(Copilot Glareshield to AFCU)
  Copilot Rudder Pedal Assembly/1(Copilot Rudder Pedal Assemby to AFCU) -> Adapter/4(Copilot Rudder Pedal Assemby to AFCU)
  Copilot Rudder Pedal Assembly/2(Copilot Rudder Pedal Control Path 1) -> Inceptor Interface Module 1 (IIM1)/4(Copilot Rudder Pedal Control Path 1)
  Pilot Rudder Pedal Assembly/1(Pilot Rudder Pedal Assembly to AFCU) -> Adapter/3(Pilot Rudder Pedal Assembly to AFCU)
  Inceptor Interface Module 3 (IIM3)/1(IIM1 to FCC1 Data Bus) -> Flight Control Computer 1 (FCC1)/3(FCC1 to IIM3 Data Bus)
  Glareshield Pilot Stick Priority Switch/2(Pilot Glareshield Priority Control Path 1) -> Inceptor Interface Module 1 (IIM1)/5(Pilot Glareshield Priority Control Path 1)
  FCC Cutout Switch/4(Flight Control Cutout Control Path 3) -> Inceptor Interface Module 3 (IIM3)/8(Flight Control Cutout Control Path 3)
  Copilot Rudder Pedal Assembly/4(Copilot Rudder Pedal Control Path 3) -> Inceptor Interface Module 3 (IIM3)/4(Copilot Rudder Pedal Control Path 3)
  Inceptor Interface Module 2 (IIM2)/3(IIM2 to FCC3 Data Bus) -> Flight Control Computer 3 (FCC3)/2(FCC3 to IIM2 Data Bus)
  In Bus Element1/1 -> Pilot Sidestick/1(Pilot Input)
  Inceptor Interface Module 2 (IIM2)/2(IIM2 to FCC2 Data Bus) -> Flight Control Computer 2 (FCC2)/2(FCC2 to IIM2 Data Bus)
  Copilot Sidestick/3(Copilot Sidestick Control Path 2) -> Inceptor Interface Module 2 (IIM2)/3(Copilot Sidestick Control Path 2)
  Inceptor Interface Module 1 (IIM1)/4(IIM to REU Data Bus) -> Remote Electronic Unit (REU)/2(REU Control Path 1)
  Pilot Sidestick/4(Pilot Sidestick to AFCU) -> Adapter/9(Pilot Sidestick to AFCU)
  Inceptor Interface Module 3 (IIM3)/3(IIM1 to FCC3 Data Bus) -> Flight Control Computer 3 (FCC3)/3(FCC3 to IIM3 Data Bus)
  Lateral Trim Switch/2(Lateral Trim Control Path 1) -> Inceptor Interface Module 1 (IIM1)/7(Lateral Trim Control Path 1)
  Glareshield Pilot Stick Priority Switch/4(Pilot Glareshield Priority Control Path 3) -> Inceptor Interface Module 3 (IIM3)/5(Pilot Glareshield Priority Control Path 3)
  In Bus Element5/1 -> Glareshield Pilot Stick Priority Switch/1(Pilot Command)
  Adapter/1(Cockpit Controls to AFCU) -> Alternate Flight Control Unit (AFCU)/1(Cockpit Controls to AFCU)
  Glareshield Pilot Stick Priority Switch/1(Pilot Glareshield to AFCU) -> Adapter/1(Pilot Glareshield to AFCU)
  In Bus Element8/1 -> Lateral Trim Switch/1(Pilot Command)
  Flight Control Computer 3 (FCC3)/1(IIM3 to AFCU Data Bus) -> Alternate Flight Control Unit (AFCU)/4(FCC3 ti AFCU)
  In Bus Element6/1 -> Glareshield Copilot Stick Priority Switch/1(Pilot Command)
  In Bus Element4/1 -> Copilot Rudder Pedal Assembly/1(Pilot Command)
  Inceptor Interface Module 3 (IIM3)/4(IIM to REU Data Bus) -> Remote Electronic Unit (REU)/4(REU Control Path 3)
  Pilot Rudder Pedal Assembly/3(Pilot Rudder Pedal Control Path 3) -> Inceptor Interface Module 3 (IIM3)/3(Pilot Rudder Pedal Control Path 3)
  In Bus Element3/1 -> Pilot Rudder Pedal Assembly/1(Pilot Command)
  Power Control Unit (PCU)/1 -> Out Bus Element3/1
  Power Control Unit (PCU)/2 -> Out Bus Element4/1
  Power Control Unit (PCU)/4 -> Out Bus Element6/1
  Power Control Unit (PCU)/3 -> Out Bus Element5/1
  Remote Electronic Unit (REU)/2(REU to PCU) -> Power Control Unit (PCU)/1

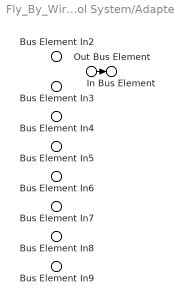
== system Fly_By_Wire_Component_Architecture/Fly By Wire Flight Control System/Adapter ==
  Bus Element In5 : Inport  PortName=Pilot Glareshield to AFCU
  Bus Element In2 : Inport  Port=2  PortName=Copilot Sidestick to AFCU
  Bus Element In3 : Inport  Port=3  PortName=Pilot Rudder Pedal Assembly to AFCU
  Bus Element In4 : Inport  Port=4  PortName=Copilot Rudder Pedal Assemby to AFCU
  Bus Element In6 : Inport  Port=5  PortName=Copilot Glareshield to AFCU
  Bus Element In7 : Inport  Port=6  PortName=FCC Cutout to AFCU
  Bus Element In8 : Inport  Port=7  PortName=Lateral Trim to AFCU
  Bus Element In9 : Inport  Port=8  PortName=FSCL to AFCU
  In Bus Element : Inport  Port=9  PortName=Pilot Sidestick to AFCU
  Out Bus Element : Outport  PortName=Cockpit Controls to AFCU
  wires:
  In Bus Element/1 -> Out Bus Element/1

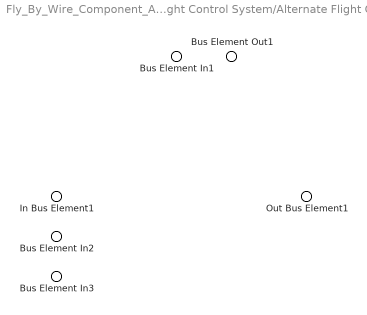
== system Fly_By_Wire_Component_Architecture/Fly By Wire Flight Control System/Alternate Flight Control Unit (AFCU) ==
  Bus Element In1 : Inport  PortName=Cockpit Controls to AFCU
  In Bus Element1 : Inport  Port=2  PortName=FCC1 to AFCU
  Bus Element In2 : Inport  Port=3  PortName=FCC2 to AFCU
  Bus Element In3 : Inport  Port=4  PortName=FCC3 ti AFCU
  Bus Element Out1 : Outport  PortName=AFCU to MCE
  Out Bus Element1 : Outport  Port=2  PortName=AFCU to PCU Data Bus

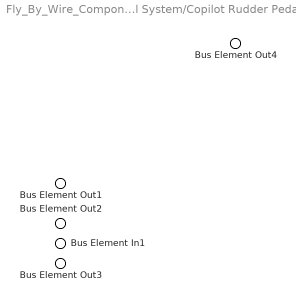
== system Fly_By_Wire_Component_Architecture/Fly By Wire Flight Control System/Copilot Rudder Pedal Assembly ==
  Bus Element In1 : Inport  PortName=Pilot Command
  Bus Element Out4 : Outport  PortName=Copilot Rudder Pedal Assemby to AFCU
  Bus Element Out1 : Outport  Port=2  PortName=Copilot Rudder Pedal Control Path 1
  Bus Element Out2 : Outport  Port=3  PortName=Copilot Rudder Pedal Control Path 2
  Bus Element Out3 : Outport  Port=4  PortName=Copilot Rudder Pedal Control Path 3

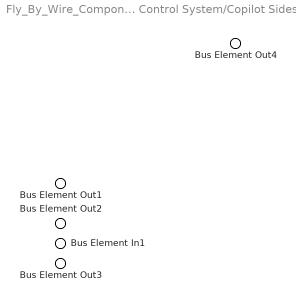
== system Fly_By_Wire_Component_Architecture/Fly By Wire Flight Control System/Copilot Sidestick ==
  Bus Element In1 : Inport  PortName=Pilot Command
  Bus Element Out4 : Outport  PortName=Copilot Sidestick to AFCU
  Bus Element Out1 : Outport  Port=2  PortName=Copilot Sidestick Control Path 1
  Bus Element Out2 : Outport  Port=3  PortName=Copilot Sidestick Control Path 2
  Bus Element Out3 : Outport  Port=4  PortName=Control Sidestick Control Path 3

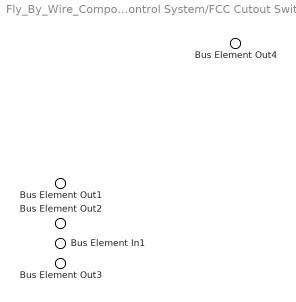
== system Fly_By_Wire_Component_Architecture/Fly By Wire Flight Control System/FCC Cutout Switch ==
  Bus Element In1 : Inport  PortName=Pilot Command
  Bus Element Out4 : Outport  PortName=FCC Cutout to AFCU
  Bus Element Out1 : Outport  Port=2  PortName=Flight Control Cutout Control Path 1
  Bus Element Out2 : Outport  Port=3  PortName=Flight Control Cutout Control Path 2
  Bus Element Out3 : Outport  Port=4  PortName=Flight Control Cutout Control Path 3

== system Fly_By_Wire_Component_Architecture/Fly By Wire Flight Control System/Flight Control Computer 1 (FCC1) ==
  In Bus Element1 : Inport  PortName=FCC1 to IIM1 Data Bus
  Bus Element In2 : Inport  Port=2  PortName=FCC1 to IIM2 Data Bus
  Bus Element In3 : Inport  Port=3  PortName=FCC1 to IIM3 Data Bus
  Out Bus Element1 : Outport  PortName=FCC to PCU Data Bus

== system Fly_By_Wire_Component_Architecture/Fly By Wire Flight Control System/Flight Control Computer 2 (FCC2) ==
  Bus Element In1 : Inport  PortName=FCC2 to IIM1 Data Bus
  Bus Element In2 : Inport  Port=2  PortName=FCC2 to IIM2 Data Bus
  Bus Element In3 : Inport  Port=3  PortName=FCC2 to IIM3 Data Bus
  Bus Element Out1 : Outport  PortName=IIM2 to AFCU Data Bus

== system Fly_By_Wire_Component_Architecture/Fly By Wire Flight Control System/Flight Control Computer 3 (FCC3) ==
  Bus Element In1 : Inport  PortName=FCC3 to IIM1 Data Bus
  Bus Element In2 : Inport  Port=2  PortName=FCC3 to IIM2 Data Bus
  Bus Element In3 : Inport  Port=3  PortName=FCC3 to IIM3 Data Bus
  Bus Element Out1 : Outport  PortName=IIM3 to AFCU Data Bus

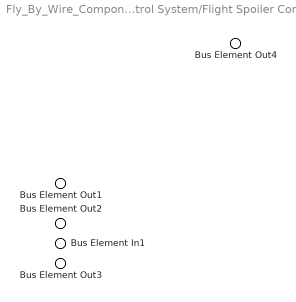
== system Fly_By_Wire_Component_Architecture/Fly By Wire Flight Control System/Flight Spoiler Control Lever (FSCL) ==
  Bus Element In1 : Inport  PortName=Pilot Command
  Bus Element Out4 : Outport  PortName=FSCL to AFCU
  Bus Element Out1 : Outport  Port=2  PortName=Spoiler Control Path 1
  Bus Element Out2 : Outport  Port=3  PortName=Spoiler Control Path 2
  Bus Element Out3 : Outport  Port=4  PortName=Spoiler Control Path 3

== system Fly_By_Wire_Component_Architecture/Fly By Wire Flight Control System/Glareshield Copilot Stick Priority Switch ==
  Bus Element In1 : Inport  PortName=Pilot Command
  Bus Element Out4 : Outport  PortName=Copilot Glareshield to AFCU
  Bus Element Out1 : Outport  Port=2  PortName=Copilot Glareshield Priority Control Path 1
  Bus Element Out2 : Outport  Port=3  PortName=Copilot Glareshield Priority Control Path 2
  Bus Element Out3 : Outport  Port=4  PortName=Copilot Glareshield Priority Control Path 3

== system Fly_By_Wire_Component_Architecture/Fly By Wire Flight Control System/Glareshield Pilot Stick Priority Switch ==
  Bus Element In1 : Inport  PortName=Pilot Command
  Bus Element Out4 : Outport  PortName=Pilot Glareshield to AFCU
  Bus Element Out1 : Outport  Port=2  PortName=Pilot Glareshield Priority Control Path 1
  Bus Element Out2 : Outport  Port=3  PortName=Pilot Glareshield Priority Control Path 2
  Bus Element Out3 : Outport  Port=4  PortName=Pilot Glareshield Priority Control Path 3

== system Fly_By_Wire_Component_Architecture/Fly By Wire Flight Control System/Ground Spoiler Control Module (GSCM) ==
  Bus Element In1 : Inport  PortName=REU to GSCM
  Out Bus Element1 : Outport  PortName=Ground Spoiler

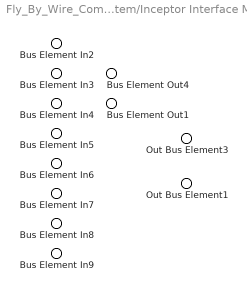
== system Fly_By_Wire_Component_Architecture/Fly By Wire Flight Control System/Inceptor Interface Module 1 (IIM1) ==
  Bus Element In2 : Inport  PortName=Pilot Sidestick Control Path 1
  Bus Element In3 : Inport  Port=2  PortName=Copilot Sidestick Control Path 1
  Bus Element In7 : Inport  Port=3  PortName=Pilot Rudder Pedal Control Path 1
  Bus Element In9 : Inport  Port=4  PortName=Copilot Rudder Pedal Control Path 1
  Bus Element In4 : Inport  Port=5  PortName=Pilot Glareshield Priority Control Path 1
  Bus Element In5 : Inport  Port=6  PortName=Copilot Glareshield Priority Control Path 1
  Bus Element In6 : Inport  Port=7  PortName=Lateral Trim Control Path 1
  Bus Element In8 : Inport  Port=8  PortName=Spoiler Control Path 1
  Out Bus Element1 : Outport  PortName=IIM1 to FCC1 Data Bus
  Bus Element Out1 : Outport  Port=2  PortName=IIM1 to FCC2 Data Bus
  Bus Element Out4 : Outport  Port=3  PortName=IIM1 to FCC3 Data Bus
  Out Bus Element3 : Outport  Port=4  PortName=IIM to REU Data Bus

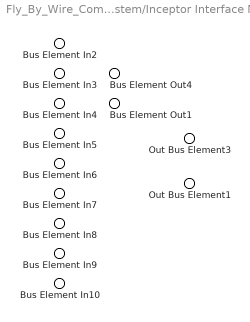
== system Fly_By_Wire_Component_Architecture/Fly By Wire Flight Control System/Inceptor Interface Module 2 (IIM2) ==
  Bus Element In3 : Inport  PortName=Pilot Sidestick Control Path 2
  Bus Element In8 : Inport  Port=2  PortName=Pilot Rudder Pedal Control Path 2
  Bus Element In2 : Inport  Port=3  PortName=Copilot Sidestick Control Path 2
  Bus Element In10 : Inport  Port=4  PortName=Copilot Rudder Pedal Control Path 2
  Bus Element In4 : Inport  Port=5  PortName=Pilot Glareshield Priority Control Path 2
  Bus Element In5 : Inport  Port=6  PortName=Copilot Glareshield Priority Control Path 2
  Bus Element In6 : Inport  Port=7  PortName=Flight Control Cutout Control Path 1
  Bus Element In7 : Inport  Port=8  PortName=Lateral Trim Control Path 2
  Bus Element In9 : Inport  Port=9  PortName=Spoiler Control Path 2
  Out Bus Element1 : Outport  PortName=IIM2 to FCC1 Data Bus
  Bus Element Out1 : Outport  Port=2  PortName=IIM2 to FCC2 Data Bus
  Bus Element Out4 : Outport  Port=3  PortName=IIM2 to FCC3 Data Bus
  Out Bus Element3 : Outport  Port=4  PortName=IIM to REU Data Bus

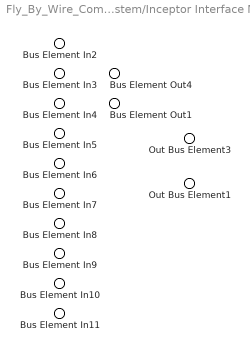
== system Fly_By_Wire_Component_Architecture/Fly By Wire Flight Control System/Inceptor Interface Module 3 (IIM3) ==
  Bus Element In3 : Inport  PortName=Pilot Sidestick Control Path 3
  Bus Element In2 : Inport  Port=2  PortName=Copilot Sidestick Control Path 3
  Bus Element In10 : Inport  Port=3  PortName=Pilot Rudder Pedal Control Path 3
  Bus Element In11 : Inport  Port=4  PortName=Copilot Rudder Pedal Control Path 3
  Bus Element In4 : Inport  Port=5  PortName=Pilot Glareshield Priority Control Path 3
  Bus Element In5 : Inport  Port=6  PortName=Copilot Glareshield Priority Control Path 3
  Bus Element In6 : Inport  Port=7  PortName=Flight Control Cutout Control Path 2
  Bus Element In7 : Inport  Port=8  PortName=Flight Control Cutout Control Path 3
  Bus Element In8 : Inport  Port=9  PortName=Lateral Trim Control Path 3
  Bus Element In9 : Inport  Port=10  PortName=Spoiler Control Path 3
  Out Bus Element1 : Outport  PortName=IIM1 to FCC1 Data Bus
  Bus Element Out1 : Outport  Port=2  PortName=IIM1 to FCC2 Data Bus
  Bus Element Out4 : Outport  Port=3  PortName=IIM1 to FCC3 Data Bus
  Out Bus Element3 : Outport  Port=4  PortName=IIM to REU Data Bus

== system Fly_By_Wire_Component_Architecture/Fly By Wire Flight Control System/Lateral Trim Switch ==
  Bus Element In1 : Inport  PortName=Pilot Command
  Bus Element Out4 : Outport  PortName=Lateral Trim to AFCU
  Bus Element Out1 : Outport  Port=2  PortName=Lateral Trim Control Path 1
  Bus Element Out2 : Outport  Port=3  PortName=Lateral Trim Control Path 2
  Bus Element Out3 : Outport  Port=4  PortName=Lateral Trim Control Path 3

== system Fly_By_Wire_Component_Architecture/Fly By Wire Flight Control System/Motor Control Electronics (MCE) ==
  Bus Element In1 : Inport  PortName=MCE to AFCU
  Bus Element Out2 : Outport  PortName=MCE to HSTA
  Bus Element Out1 : Outport  Port=2  PortName=MCE to REU

== system Fly_By_Wire_Component_Architecture/Fly By Wire Flight Control System/Pilot Rudder Pedal Assembly ==
  Bus Element In1 : Inport  PortName=Pilot Command
  Bus Element Out3 : Outport  PortName=Pilot Rudder Pedal Assembly to AFCU
  Bus Element Out1 : Outport  Port=2  PortName=Pilot Rudder Pedal Control Path 1
  Bus Element Out4 : Outport  Port=3  PortName=Pilot Rudder Pedal Control Path 3
  Bus Element Out2 : Outport  Port=4  PortName=Pilot Rudder Pedal Control Path 2

== system Fly_By_Wire_Component_Architecture/Fly By Wire Flight Control System/Pilot Sidestick ==
  Bus Element In1 : Inport  PortName=Pilot Input
  Bus Element Out1 : Outport  PortName=Pilot Sidestick Control Path 1
  Bus Element Out2 : Outport  Port=2  PortName=Pilot Sidestick Control Path 2
  Bus Element Out3 : Outport  Port=3  PortName=Pilot Sidestick Control Path 3
  Out Bus Element1 : Outport  Port=4  PortName=Pilot Sidestick to AFCU

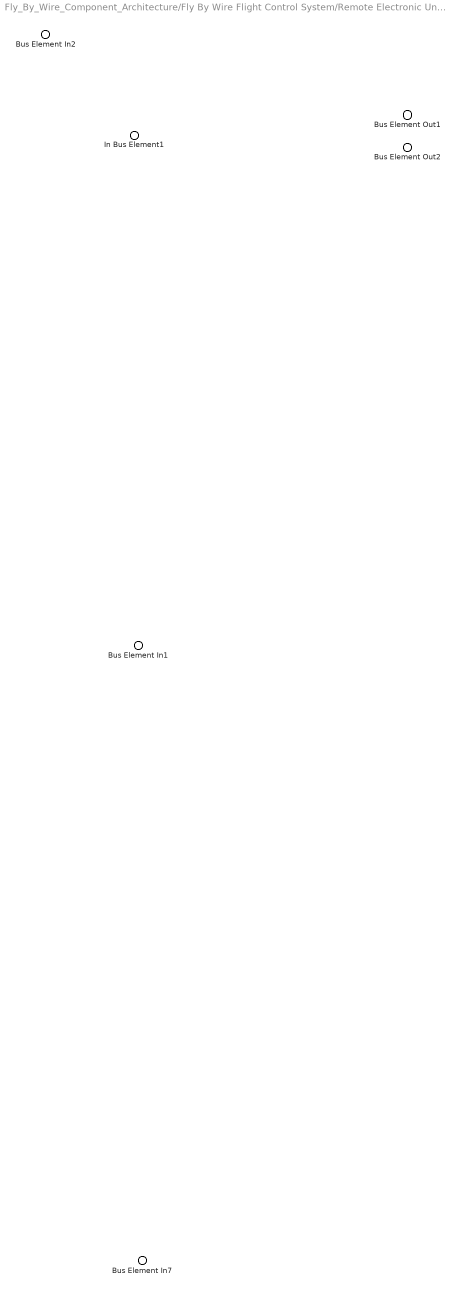
== system Fly_By_Wire_Component_Architecture/Fly By Wire Flight Control System/Remote Electronic Unit (REU) ==
  Bus Element In2 : Inport  PortName=REU to MCE
  In Bus Element1 : Inport  Port=2  PortName=REU Control Path 1
  Bus Element In1 : Inport  Port=3  PortName=REU Control Path 2
  Bus Element In7 : Inport  Port=4  PortName=REU Control Path 3
  Bus Element Out1 : Outport  PortName=REU to GSCM
  Bus Element Out2 : Outport  Port=2  PortName=REU to PCU
